simulink model "PV_vsi_sf"  (R2017a)
settings: Solver=ode4  StartTime=0.0  StopTime=6  FixedStep=1e-4  RelTol=1e-3
InitFcn:
  | SimulinkInit
values from neighbouring files (symbols this model uses):
  C3 = 610e-6    (= 0.00061)    [Parametros_Sistema.m]    (also in SimulinkInit.m; SimulinkInit_linea_transmision.m; sistema.m)
  L3 = 5e-3    (= 0.005)    [Parametros_Sistema.m]    (also in SimulinkInit.m = 0.03; SimulinkInit_linea_transmision.m; sistema.m)
  R3 = 1e-3    (= 0.001)    [Parametros_Sistema.m]    (also in SimulinkInit.m; SimulinkInit_linea_transmision.m; sistema.m)
settings Model: Creator=carma  LastModifiedBy=Administrador
settings OptimizationCC: DefaultParameterBehavior=Inlined  PassReuseOutputArgsAs=Individual arguments
settings DebuggingCC: ParameterTunabilityLossMsg=error
settings SFSimCC: MATLABDynamicMemAlloc=off
settings RTWCC: SystemTargetFile=ert.tlc  TemplateMakefile=ert_default_tmf  Description=Embedded Coder  GenerateReport=on  IncludeHyperlinkInReport=on  LaunchReport=on  GenerateTraceInfo=on  GenerateTraceReport=on  GenerateTraceReportSl=on  GenerateTraceReportSf=on  GenerateTraceReportEml=on
settings CodeAppCC: ForceParamTrailComments=on  IgnoreCustomStorageClasses=off  OperatorAnnotations=on  SimulinkDataObjDesc=on  SFDataObjDesc=on  MATLABFcnDesc=on  InsertBlockDesc=on  MATLABSourceComments=on
settings ERTTargetCC: TargetLangStandard=C99 (ISO)  GenerateSampleERTMain=on  SupportContinuousTime=on  InlinedParameterPlacement=NonHierarchical  ERTCustomFileTemplate=example_file_process.tlc

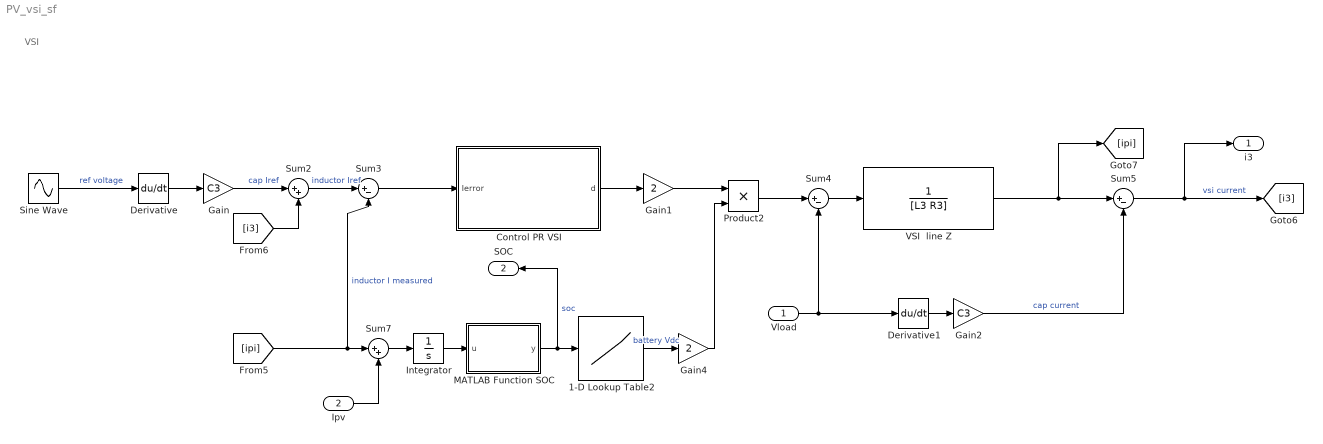
== system PV_vsi_sf ==
  note: VSI
  Vload : Inport
  Ipv : Inport  Port=2
  1-D Lookup Table2 : Lookup_n-D  NumberOfTableDimensions=1  BreakpointsForDimension1=[0 10 20 30 40 50 70 80 100]  Table=[0 10 200 500 800 1000 1140 1150 1200]  InternalRulePriority=Speed  RndMeth=Simplest  InputSameDT=on
  Control PR VSI : Subsystem
  Derivative : Derivative
  Derivative1 : Derivative
  Gain : Gain  Gain=C3
  Gain1 : Gain  Gain=2
  Gain2 : Gain  Gain=C3
  Gain4 : Gain  Gain=2
  Integrator : Integrator  LimitOutput=on  UpperSaturationLimit=1  LowerSaturationLimit=0
  "MATLAB Function SOC " : MATLAB Function  TreatAsAtomicUnit=on
  Product2 : Product
  Sine Wave : Sin  Amplitude=170  Frequency=2*pi*60  SampleTime=0
  Sum2 : Sum  Inputs=|++
  Sum3 : Sum  Inputs=|+-
  Sum4 : Sum  Inputs=|+-
  Sum5 : Sum  Inputs=|+-
  Sum7 : Sum  Inputs=|++
  VSI  line Z : TransferFcn  Denominator=[L3 R3]
  i3 : Outport
  SOC : Outport  Port=2
  wires:
  Sine Wave/1 -> Derivative/1  "ref voltage"
  Derivative/1 -> Gain/1
  Gain/1 -> Sum2/1  "cap Iref"
  Sum2/1 -> Sum3/1  "inductor Iref"
  Sum3/1 -> Control PR VSI/1(Ierror)
  Control PR VSI/1(d) -> Gain1/1
  Gain1/1 -> Product2/1
  Product2/1 -> Sum4/1
  Vload/1 -> Sum4/2, Derivative1/1
  Derivative1/1 -> Gain2/1
  Sum4/1 -> VSI  line Z/1
  VSI  line Z/1 -> [ipi], Sum5/1
  Gain2/1 -> Sum5/2  "cap current"
  Sum5/1 -> i3/1, [i3]  "vsi current"
  [ipi] -> Sum7/1, Sum3/2  "inductor I measured"
  [i3] -> Sum2/2
  Integrator/1 -> "MATLAB Function SOC "/1(u)
  "MATLAB Function SOC "/1(y) -> SOC/1, 1-D Lookup Table2/1  "soc"
  1-D Lookup Table2/1 -> Gain4/1  "battery Vdc"
  Gain4/1 -> Product2/2
  Sum7/1 -> Integrator/1
  Ipv/1 -> Sum7/2

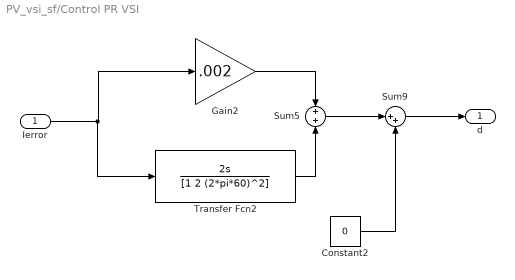
== system PV_vsi_sf/Control PR VSI ==
  Ierror : Inport
  Constant2 : Constant  Value=0
  Gain2 : Gain  Gain=.002
  Sum5 : Sum  Inputs=+|+
  Sum9 : Sum  Inputs=|++
  Transfer Fcn2 : TransferFcn  Numerator=[2 0]  Denominator=[1 2 (2*pi*60)^2]
  d : Outport
  wires:
  Constant2/1 -> Sum9/2
  Sum5/1 -> Sum9/1
  Transfer Fcn2/1 -> Sum5/2
  Gain2/1 -> Sum5/1
  Ierror/1 -> Transfer Fcn2/1, Gain2/1
  Sum9/1 -> d/1

== matlab function PV_vsi_sf/MATLAB Function SOC  ==
  data: u input; y output
function y = fcn(u)

y = -0.03536*u+100;
